simulink model "FullHopper_alt"  (R2020a)
settings: Solver=ode4  StartTime=0  StopTime=10  FixedStep=0.0005  RelTol=1e-7  AbsTol=1e-9  EnableMultiTasking=on
model workspace (MAT data in the model file):
  Mass = 35
  T_stim = 0.4
  dpMass0 = -0.0171675
  gravity = 9.81
  k_shoe = 20000
  thickness = 0.03
settings Model: OrderedModelArguments=off  Creator=Laksh  LastModifiedBy=jmei13
settings SolverCC: AutoScaleAbsTol=off  MaxConsecutiveMinStep=10  AlgebraicLoopSolver=LineSearch
settings DataIOCC: SaveFormat=StructureWithTime  SignalLogging=off
settings OptimizationCC: LifeSpan=inf
settings DebuggingCC: ReadBeforeWriteMsg=DisableAll  WriteAfterWriteMsg=DisableAll  WriteAfterReadMsg=DisableAll  AlgebraicLoopMsg=none  MultiTaskDSMMsg=none  SFUnexpectedBacktrackingDiag=warning  SFNoUnconditionalDefaultTransitionDiag=warning  SFExecutionAtInitializationDiag=none  ArithmeticOperatorsInVariantConditions=warning
settings ModelReferenceCC: UpdateModelReferenceTargets=IfOutOfDate  ModelReferenceMinAlgLoopOccurrences=on
settings SFSimCC: SFSimEcho=off  SimUseLocalCustomCode=off  CustomCodeUndefinedFunction=UseInterfaceOnly
settings RTWCC: RTWUseLocalCustomCode=off
settings CodeAppCC: StateflowObjectComments=on
settings GRTTargetCC: TargetLangStandard=C89/C90 (ANSI)
settings ConfigComp: CovMetricSettings=dw  CovHtmlReporting=on  CovSaveCumulativeToWorkspaceVar=on  CovSaveSingleToWorkspaceVar=on  CovExternalEMLEnable=off

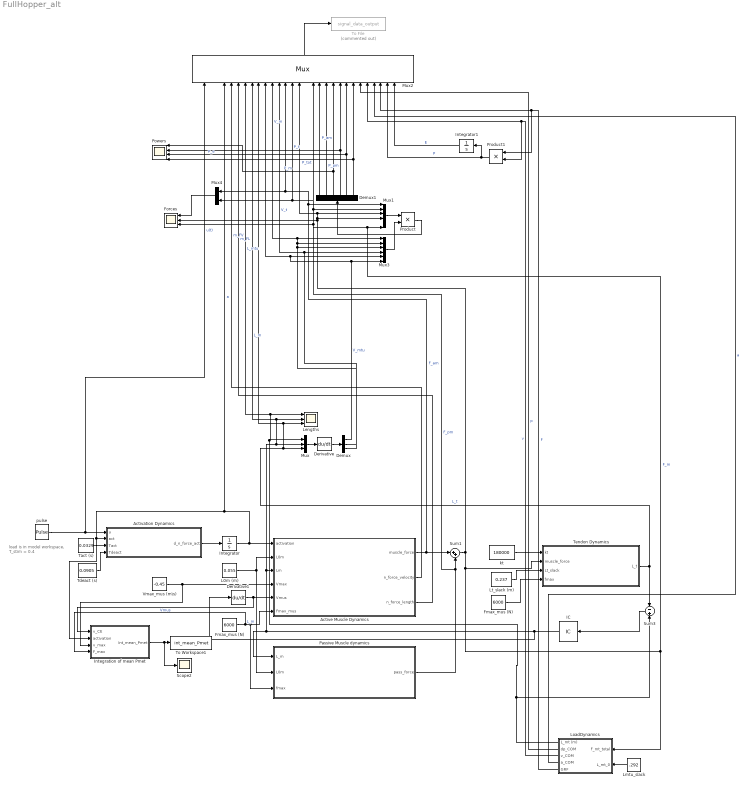
== system FullHopper_alt ==
  note: load is in model workspace,
      | T_stim = 0.4
  Activation Dynamics : MATLAB Function  TreatAsAtomicUnit=on
  Active Muscle Dynamics : MATLAB Function
  Demux : Demux  Outputs=3
  Demux1 : Demux  Outputs=6
  Derivative : Derivative
  Derivative1 : Derivative
  Fmax_mus (N) : Constant  Value=6000
  "Fmax_mus (N) " : Constant  Value=6000
  Forces : Scope  NumInputPorts=3
  IC : InitialCondition  Value=0.055
  Integration of mean Pmet : Subsystem
  Integrator : Integrator
  Integrator1 : Integrator
  L0m (m) : Constant  Value=0.055
  Lengths : Scope  NumInputPorts=3
  Lmtu_slack : Constant  Value=.292
  LoadDynamics : Subsystem
  Lt_slack (m) : Constant  Value=0.237
  Mux : Mux  Inputs=3
  Mux1 : Mux  Inputs=6
  Mux2 : Mux  Inputs=30
      settings: DisplayOption=signals
  Mux3 : Mux  Inputs=6
  Mux4 : Mux  Inputs=2
  Passive Muscle dynamics : MATLAB Function
  Powers : Scope  NumInputPorts=4
  Product : Product
  Product1 : Product
  Scope2 : Scope
  Sum1 : Sum  Inputs=|++
  Sum3 : Sum  Inputs=-|+
  Tact (s) : Constant  Value=0.0329  VectorParams1D=off
  Tdeact (s) : Constant  Value=0.0905
  Tendon Dynamics : MATLAB Function
  To File : ToFile  Commented=on  Filename=signal_data_output  MatrixName=data  SaveFormat=Timeseries
  To Workspace1 : ToWorkspace  VariableName=int_mean_Pmet  SaveFormat=Timeseries  SampleTime=-1
  Vmax_mus (m\s) : Constant  Value=-0.45
  kt : Constant  Value=180000
  pulse : DiscretePulseGenerator  PulseType=Time based  Period=T_stim  PulseWidth=50
  wires:
  Activation Dynamics/1(d_n_force_act) -> Integrator/1
  Tact (s)/1 -> Activation Dynamics/3(Tact)
  Tdeact (s)/1 -> Activation Dynamics/4(Tdeact)
  L0m (m)/1 -> Active Muscle Dynamics/2(L0m), Passive Muscle dynamics/2(L0m)  "L_m"
  Passive Muscle dynamics/1(pass_force) -> Mux1/2, Mux4/2, Mux2/14, Sum1/2  "F_pm"
  Sum1/1 -> Mux1/4, Mux1/3, Mux2/15, Forces/2, LoadDynamics/1(F_mt_total), Mux1/6, Forces/3, Mux2/17, Tendon Dynamics/2(muscle_force)  "F_m"
  Lt_slack (m)/1 -> Tendon Dynamics/3(Lt_slack)
  kt/1 -> Tendon Dynamics/1(kt)
  LoadDynamics/1(L_mt (m)) -> Sum3/2, Lengths/1, Mux2/7, Mux/1  "L_mtu"
  Active Muscle Dynamics/1(muscle_force) -> Sum1/1, Mux1/1, Mux4/1, Mux2/13  "F_am"
  Mux2/1 -> To File/1
  Lmtu_slack/1 -> LoadDynamics/2(L_mt_0)
  Active Muscle Dynamics/2(n_force_velocity) -> Mux2/5  "m_FV"
  Active Muscle Dynamics/3(n_force_length) -> Mux2/6  "m_FL"
  Mux/1 -> Derivative/1
  Derivative/1 -> Demux/1
  Demux/1 -> Mux3/5, Mux2/10, Mux3/6  "V_mtu"
  Demux/2 -> Mux3/3, Mux3/2, Mux3/1, Mux2/11  "V_m"
  Demux/3 -> Mux3/4, Mux2/12  "V_t"
  Mux1/1 -> Product/1
  Mux3/1 -> Product/2
  Product/1 -> Demux1/1
  Demux1/1 -> Mux2/18  "P_am"
  Demux1/2 -> Mux2/19  "P_pm"
  Demux1/3 -> Mux2/20, Powers/1  "P_m"
  Demux1/4 -> Mux2/21, Powers/2  "P_t"
  Demux1/5 -> Mux2/22, Powers/3  "P_e"
  Demux1/6 -> Mux2/23, Powers/4  "P_tot"
  LoadDynamics/2(dp_COM) -> Mux2/24  "p"
  LoadDynamics/3(v_COM) -> Product1/2, Mux2/25  "v"
  LoadDynamics/4(a_COM) -> Mux2/26  "a"
  LoadDynamics/5(GRF) -> Product1/1, Mux2/27  "F"
  Product1/1 -> Mux2/28, Integrator1/1  "P"
  Integrator1/1 -> Mux2/29  "E"
  "Fmax_mus (N) "/1 -> Tendon Dynamics/4(fmax)
  Tendon Dynamics/1(L_t) -> Lengths/3, Mux2/9, Mux/3, Sum3/1  "L_t"
  Sum3/1 -> IC/1
  IC/1 -> Derivative1/1, Passive Muscle dynamics/1(L_m), Mux/2, Lengths/2, Mux2/8, Active Muscle Dynamics/3(Lm)  "L_m"
  Mux4/1 -> Forces/1
  pulse/1 -> Mux2/1, Activation Dynamics/1(u)  "u(t)"
  Vmax_mus (m\s)/1 -> Integration of mean Pmet/3(v_max), Active Muscle Dynamics/4(Vmax)
  Derivative1/1 -> Integration of mean Pmet/1(v_CE), Active Muscle Dynamics/5(Vmus)  "Vmus"
  Integration of mean Pmet/1(Int_mean_Pmet) -> To Workspace1/1, Scope2/1
  Integrator/1 -> Active Muscle Dynamics/1(activation), Integration of mean Pmet/2(activation), Activation Dynamics/2(act), Mux2/4  "a"
  Fmax_mus (N)/1 -> Integration of mean Pmet/4(F_max), Passive Muscle dynamics/3(fmax), Active Muscle Dynamics/6(Fmax_mus)

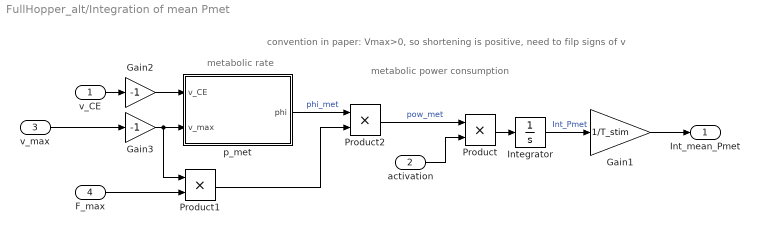
== system FullHopper_alt/Integration of mean Pmet ==
  note: convention in paper: Vmax>0, so shortening is positive, need to filp signs of v
  note: metabolic power consumption
  note: metabolic rate
  v_CE : Inport
  activation : Inport  Port=2
  v_max : Inport  Port=3
  F_max : Inport  Port=4
  Gain1 : Gain  Gain=1/T_stim
  Gain2 : Gain  Gain=-1
  Gain3 : Gain  Gain=-1
  Integrator : Integrator
  Product : Product
  Product1 : Product
  Product2 : Product
  p_met : MATLAB Function  TreatAsAtomicUnit=on
  Int_mean_Pmet : Outport
  wires:
  v_CE/1 -> Gain2/1
  activation/1 -> Product/2
  Product/1 -> Integrator/1
  Integrator/1 -> Gain1/1  "Int_Pmet"
  Product2/1 -> Product/1  "pow_met"
  p_met/1(phi) -> Product2/1  "phi_met"
  Gain3/1 -> Product1/1, p_met/2(v_max)
  Gain1/1 -> Int_mean_Pmet/1
  Gain2/1 -> p_met/1(v_CE)
  v_max/1 -> Gain3/1
  F_max/1 -> Product1/2
  Product1/1 -> Product2/2

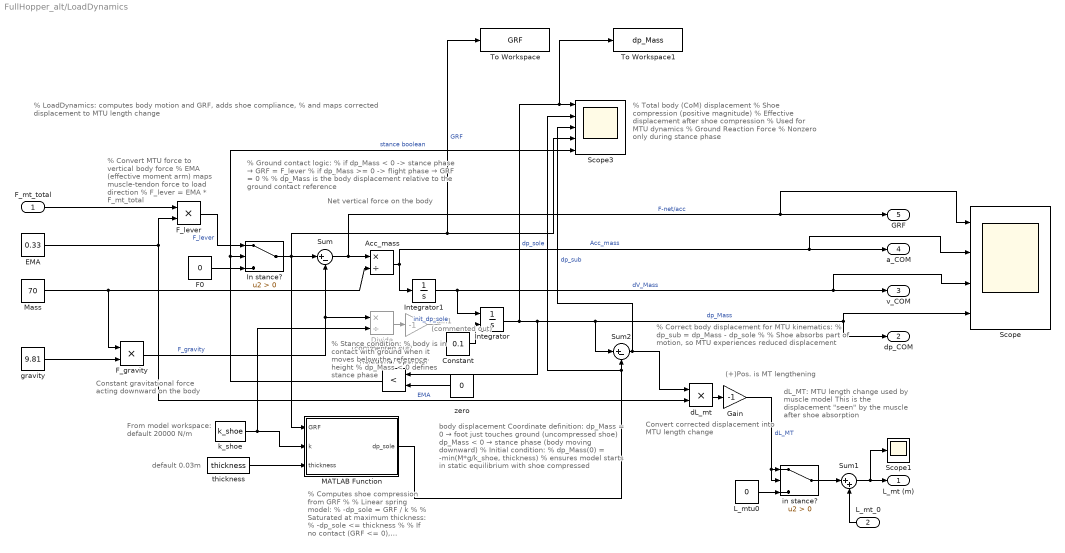
== system FullHopper_alt/LoadDynamics ==
  note: % Total body (CoM) displacement
      |
      | % Shoe compression (positive magnitude)
      |
      | % Effective displacement after shoe compression
      | % Used for MTU dynamics
      |
      | % Ground Reaction Force
      | % Nonzero only during stance phase
  note: % LoadDynamics: computes body motion and GRF, adds shoe compliance,
      | % and maps corrected displacement to MTU length change
  note: dL_MT:
      | MTU length change used by muscle model
      | This is the displacement "seen" by the muscle after shoe absorption
  note: Convert corrected displacement into MTU length change
  note: % Correct body displacement for MTU kinematics:
      | % dp_sub = dp_Mass - dp_sole
      | %
      | % Shoe absorbs part of motion, so MTU experiences reduced displacement
  note: % Computes shoe compression from GRF
      | %
      | % Linear spring model:
      | % -dp_sole = GRF / k
      | %
      | % Saturated at maximum thickness:
      | % -dp_sole <= thickness
      | %
      | % If no contact (GRF <= 0), compression = 0
  note: body displacement
      | Coordinate definition:
      | dp_Mass = 0 → foot just touches ground (uncompressed shoe)
      | dp_Mass < 0 → stance phase (body moving downward)
      |
      | % Initial condition:
      | % dp_Mass(0) = -min(M*g/k_shoe, thickness)
      | % ensures model starts in static equilibrium with shoe compressed
  note: Net vertical force on the body
  note: % Stance condition:
      | % body is in contact with ground when it moves below the reference height
      | % dp_Mass < 0 defines stance phase
  note: % Ground contact logic:
      | % if dp_Mass < 0 -> stance phase → GRF = F_lever
      | % if dp_Mass >= 0 -> flight phase → GRF = 0
      | %
      | % dp_Mass is the body displacement relative to the ground contact reference
  note: Constant gravitational force acting downward on the body
  note: From model workspace:
      | default 20000 N/m
  note: (+)Pos. is MT
      | lengthening
  note: default 0.03m
  note: % Convert MTU force to vertical body force
      | % EMA (effective moment arm) maps muscle-tendon force to load direction
      | % F_lever = EMA * F_mt_total
  F_mt_total : Inport
  L_mt_0 : Inport  Port=2
  Acc_mass : Product  Inputs=*/
  Constant : Constant  Value=0.1
  Divide : Product  Commented=on  Inputs=*/
  EMA : Constant  Value=0.33
  F0 : Constant  Value=0
  F_gravity : Product  RndMeth=Zero
  F_lever : Product  RndMeth=Zero
  Gain : Gain  Gain=-1
  Gain1 : Gain  Commented=on  Gain=-1
  In stance? : Switch  Criteria=u2 > Threshold
  Integrator : Integrator  InitialConditionSource=external  InitialCondition=dpMass0
  Integrator1 : Integrator
  L_mtu0 : Constant  Value=0
  MATLAB Function : MATLAB Function  TreatAsAtomicUnit=on
  Mass : Constant  Value=70
  Relational Operator : RelationalOperator  Operator=<  OutDataTypeStr=boolean  RndMeth=Simplest
  Scope : Scope  NumInputPorts=4
  Scope1 : Scope
  Scope3 : Scope  NumInputPorts=5
  Sum : Sum  Inputs=|+-
  Sum1 : Sum  Inputs=|++
  Sum2 : Sum  Inputs=|+-
  To Workspace : ToWorkspace  VariableName=GRF  SaveFormat=Timeseries  SampleTime=-1
  To Workspace1 : ToWorkspace  VariableName=dp_Mass  SaveFormat=Timeseries  SampleTime=-1
  dL_mt : Product  RndMeth=Zero
  gravity : Constant  Value=9.81
  "in stance? " : Switch  Criteria=u2 > Threshold
  k_shoe : Constant  Value=k_shoe
  thickness : Constant  Value=thickness
  zero : Constant  Value=0
  L_mt (m) : Outport
  dp_COM : Outport  Port=2
  v_COM : Outport  Port=3
  a_COM : Outport  Port=4
  GRF : Outport  Port=5
  wires:
  Integrator1/1 -> Integrator/1, Scope/3, v_COM/1  "dV_Mass"
  Sum1/1 -> Scope1/1, L_mt (m)/1
  L_mt_0/1 -> Sum1/2
  Acc_mass/1 -> Scope/2, a_COM/1, Integrator1/1  "Acc_mass"
  F0/1 -> In stance?/3
  Sum/1 -> Scope/1, GRF/1, Acc_mass/1  "F-net/acc"
  F_mt_total/1 -> F_lever/1
  Gain/1 -> "in stance? "/1, "in stance? "/2  "dL_MT"
  dL_mt/1 -> Gain/1
  F_lever/1 -> In stance?/1  "F_lever"
  Integrator/1 -> Relational Operator/1, Sum2/1, Scope/4, dp_COM/1, To Workspace1/1, Scope3/1  "dp_Mass"
  F_gravity/1 -> Divide/1, Sum/2  "F_gravity"
  EMA/1 -> F_lever/2, dL_mt/2  "EMA"
  gravity/1 -> F_gravity/2
  Mass/1 -> F_gravity/1, Acc_mass/2
  L_mtu0/1 -> "in stance? "/3
  In stance?/1 -> Sum/1, To Workspace/1, Scope3/4, MATLAB Function/1(GRF)  "GRF"
  "in stance? "/1 -> Sum1/1
  MATLAB Function/1(dp_sole) -> Scope3/2, Sum2/2  "dp_sole"
  Sum2/1 -> Scope3/3, dL_mt/1  "dp_sub"
  zero/1 -> Relational Operator/2
  Relational Operator/1 -> In stance?/2, Scope3/5  "stance boolean"
  k_shoe/1 -> Divide/2, MATLAB Function/2(k)
  thickness/1 -> MATLAB Function/3(thickness)
  Divide/1 -> Gain1/1
  Gain1/1 -> ?  "init_dp_sole"
  Constant/1 -> Integrator/2

== matlab function FullHopper_alt/LoadDynamics/MATLAB Function ==
  data: GRF input; dp_sole output; k input; thickness input
function dp_sole = shoe_disp(GRF,k,thickness)
% Computes shoe (sole) compression based on ground reaction force (GRF)
% This compression is subtracted from CoM displacement:
%   dp_sub = dp_Mass - dp_sole
% Inputs:
%   GRF       - Ground Reaction Force (N)
%   k         - Shoe stiffness (N/m)
%   thickness - Maximum allowable compression of the sole (m)
%
% Output:
%   dp_sole   - Displacement/Compression of the shoe sole (m, negative value)
%   taken as negative to match the displacement coordinates like dp_COM.

% Case 1: No contact (flight phase)
% If GRF is zero or negative, the foot is not in contact with the ground
% → no compression in the shoe
if GRF <= 0
    dp_sole = 0;

else
    % Case 2: Foot is in contact (stance phase)
    
    % Compute linear spring compression using Hooke's Law:
    %   F = kx  →  x = F/k
    x = GRF / k;
    
    % Limit compression to the physical thickness of the sole
    % This prevents unrealistic "over-compression"
    if x > thickness
        x = thickness;
    end
    
    % Output compression
    % Note: dp_sole is defined as a positive quantity (magnitude of compression)
    dp_sole = x;
end

% reflect the sign to match displacement convention: 
% upwards is positive

dp_sole = -dp_sole;

== matlab function FullHopper_alt/Active Muscle Dynamics ==
  data: activation input; L0m input; Lm input; Vmax input; Vmus input; Fmax_mus input; muscle_force output; n_force_velocity output; n_force_length output
function [muscle_force, n_force_velocity, n_force_length]  =...
    muscle_dynamics(activation,L0m,Lm,Vmax,Vmus,Fmax_mus)
%#codegen

    %Hill Type Muscle F-V relationship.  Returns a normalized force-velocity value
    if (Vmus<Vmax)
        n_force_velocity=0;
    else
        if (Vmus >= Vmax && Vmus < 0)
            n_force_velocity = ((1-(Vmus/Vmax))/(1+(Vmus/0.17/Vmax)));
        else
            n_force_velocity =(1.8-0.8*((1+(Vmus/Vmax))/(1-7.56*Vmus/0.17/Vmax)));
        end
    end
    
    %Active muscle F-L relationships.  Returns a normalized F-L value

    a = 3.1108;
    b = .8698;
    s = .3914;

    if Lm < 0
        Lm = 0;
    end

    n_force_length = exp(-(abs(((Lm/L0m)^b-1)/s))^a);

    %Total active force of muscle based on normalized F-V and F-L relationships
    muscle_force = Fmax_mus* activation * n_force_velocity * n_force_length;
end

== matlab function FullHopper_alt/Tendon Dynamics ==
  data: kt input; L_t output; muscle_force input; Lt_slack input; fmax input
function L_t = L_tendon(kt,muscle_force,Lt_slack,fmax)
%#codegen

%Total tendon length
%kt_comp = @(fm) 1./(kt*(1+(0.9./((-exp((20*fm)./fmax))))));
dL_t = ((muscle_force + (fmax*log((-9*exp(-(20*muscle_force)/fmax)) + 10))/20)/kt);
L_t = dL_t + Lt_slack ;

end

== matlab function FullHopper_alt/Activation Dynamics ==
  data: u input; d_n_force_act output; act input; Tact input; Tdeact input
function d_n_force_act = d_n_force_act(u,act,Tact,Tdeact)
%#codegen    
%Rate of change of activation
    B=Tact/Tdeact;
    d_n_force_act= u/Tact - (1/Tact*(B+(1-B)*u))*act;
end

== matlab function FullHopper_alt/Passive Muscle dynamics ==
  data: pass_force output; L_m input; L0m input; fmax input
function pass_force = pmuscle_dynamics(L_m, L0m,fmax)
%#codegen
%passive CE F_L taken from Rubenson et. al.

%Passive muscle force
A = 2.38*10^(-2);
b = 5.31;

if L_m > 0    
    pass_force= fmax*A*exp(b*((L_m/L0m)-1));
else
    pass_force=0;
end


end

== matlab function FullHopper_alt/Integration of mean Pmet/p_met ==
  data: v_CE input; phi output; v_max input
function phi = p_met(v_CE, v_max)

if v_CE<0
    phi = 0.01 - 0.11*(v_CE/v_max) + 0.06*exp(23*v_CE/v_max);
else
    phi = 0.23 - 0.16*exp(-8*v_CE/v_max);
end
